simulink subsystem "ADC_Block"  (R2024b)
settings: Solver=VariableStepAuto  StartTime=0.0  StopTime=10.0  RelTol=1e-3
undefined symbols (not defined in the file or in its folder): circularBufferSize, samplingTime
settings Model: Creator=JesseJabezArendse  LastModifiedBy=JesseJabezArendse
settings RTWCC: GPUComputeCapability=3.5

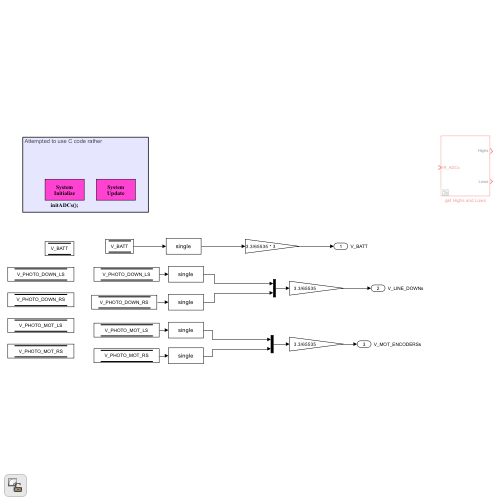
[thumbnail: Simulink's stored preview of the top-level diagram]
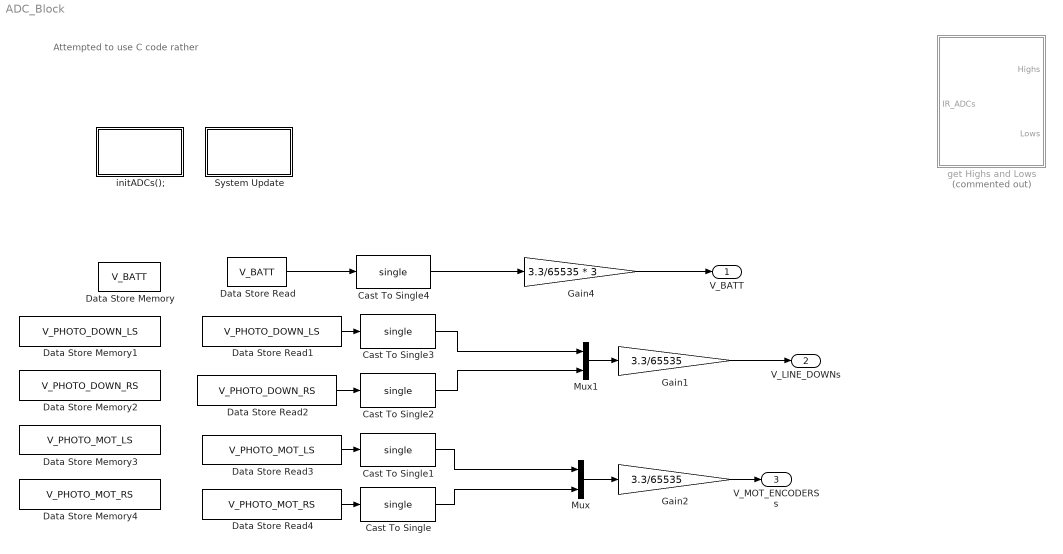
== system ADC_Block ==
  note: Attempted to use C code rather
  Cast To Single{,1..4} (5 alike) : DataTypeConversion  OutDataTypeStr=single  SaturateOnIntegerOverflow=off  RndMeth=Floor
  Data Store Memory : DataStoreMemory  DataStoreName=V_BATT  WriteAfterWriteMsg=warning  ShowAdditionalParam=off  OutDataTypeStr=uint16  Dimensions=1
  Data Store Memory1 : DataStoreMemory  DataStoreName=V_PHOTO_DOWN_LS  WriteAfterWriteMsg=warning  ShowAdditionalParam=off  OutDataTypeStr=uint16  Dimensions=1
  Data Store Memory2 : DataStoreMemory  DataStoreName=V_PHOTO_DOWN_RS  WriteAfterWriteMsg=warning  ShowAdditionalParam=off  OutDataTypeStr=uint16  Dimensions=1
  Data Store Memory3 : DataStoreMemory  DataStoreName=V_PHOTO_MOT_LS  WriteAfterWriteMsg=warning  ShowAdditionalParam=off  OutDataTypeStr=uint16  Dimensions=1
  Data Store Memory4 : DataStoreMemory  DataStoreName=V_PHOTO_MOT_RS  WriteAfterWriteMsg=warning  ShowAdditionalParam=off  OutDataTypeStr=uint16  Dimensions=1
  Data Store Read : DataStoreRead  DataStoreName=V_BATT  IndexOptions=Index vector (dialog)  Indices=1  OutputSizes=1
  Data Store Read1 : DataStoreRead  DataStoreName=V_PHOTO_DOWN_LS  IndexOptions=Index vector (dialog)  Indices=1  OutputSizes=1
  Data Store Read2 : DataStoreRead  DataStoreName=V_PHOTO_DOWN_RS  IndexOptions=Index vector (dialog)  Indices=1  OutputSizes=1
  Data Store Read3 : DataStoreRead  DataStoreName=V_PHOTO_MOT_LS  IndexOptions=Index vector (dialog)  Indices=1  OutputSizes=1
  Data Store Read4 : DataStoreRead  DataStoreName=V_PHOTO_MOT_RS  IndexOptions=Index vector (dialog)  Indices=1  OutputSizes=1
  Gain1 : Gain  Gain=3.3/65535
  Gain2 : Gain  Gain=3.3/65535
  Gain4 : Gain  Gain=3.3/65535 * 3
  Mux : Mux  Inputs=2
  Mux1 : Mux  Inputs=2
  System Update : Subsystem  mask(System Update){ShowInLibBrowser=0}
      mask prompts: ShowInLibBrowser "Simulink:masks:CustCodeMaskParam1_MP"
      settings: CopyFcn=cccopyfcn(gcb)  OpenFcn=ccopenfcn('System Update Function')
      mask Help: eval('feval(''rtwprivate'',''rtwhelpview'',''rtw_sys_update_block'')');
      mask Display: disp('System\nUpdate');
  get Highs and Lows : Subsystem  Commented=on
  initADCs(); : Subsystem  mask(System Initialize){ShowInLibBrowser=0}
      mask prompts: ShowInLibBrowser "Simulink:masks:CustCodeMaskParam1_MP"
      settings: CopyFcn=cccopyfcn(gcb)  OpenFcn=ccopenfcn('System Initialize Function')
      mask Help: eval('feval(''rtwprivate'',''rtwhelpview'',''rtw_sys_initialize_block'')');
      mask Display: disp('System\nInitialize');
  V_BATT : Outport
  V_LINE_DOWNs : Outport  Port=2
  V_MOT_ENCODERSs : Outport  Port=3
  wires:
  Mux1/1 -> Gain1/1
  Gain4/1 -> V_BATT/1
  Mux/1 -> Gain2/1
  Data Store Read/1 -> Cast To Single4/1
  Data Store Read3/1 -> Cast To Single1/1
  Data Store Read4/1 -> Cast To Single/1
  Data Store Read1/1 -> Cast To Single3/1
  Data Store Read2/1 -> Cast To Single2/1
  Gain1/1 -> V_LINE_DOWNs/1
  Gain2/1 -> V_MOT_ENCODERSs/1
  Cast To Single/1 -> Mux/2
  Cast To Single1/1 -> Mux/1
  Cast To Single2/1 -> Mux1/2
  Cast To Single3/1 -> Mux1/1
  Cast To Single4/1 -> Gain4/1

== system ADC_Block/System Update ==

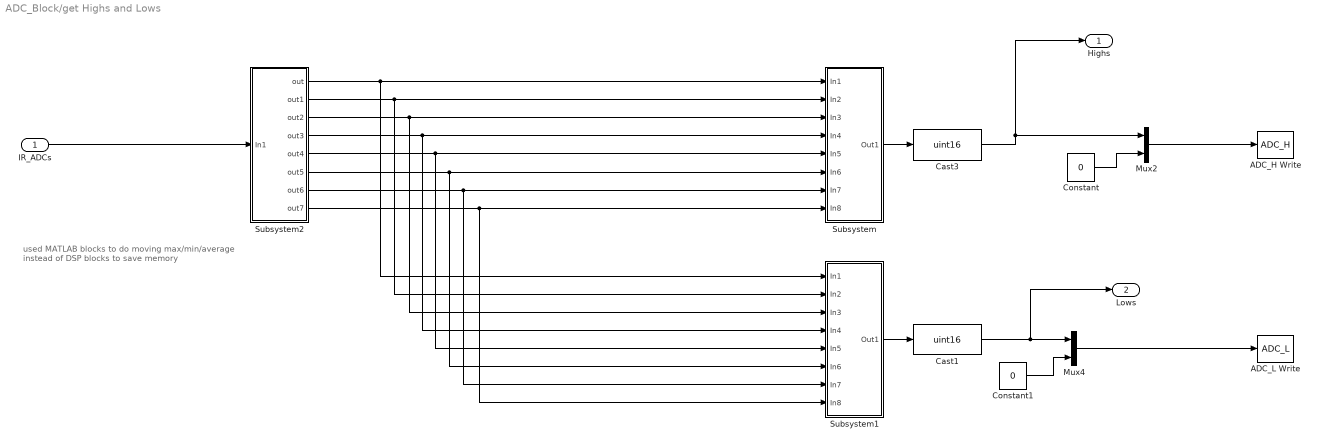
== system ADC_Block/get Highs and Lows ==
  note: used MATLAB blocks to do moving max/min/average
      | instead of DSP blocks to save memory
  IR_ADCs : Inport  PortDimensions=8  SampleTime=samplingTime
  ADC_H Write : DataStoreWrite  DataStoreName=ADC_H  SampleTime=samplingTime  IndexOptions=Index vector (dialog)  Indices=1  OutputSizes=1
  ADC_L Write : DataStoreWrite  DataStoreName=ADC_L  SampleTime=samplingTime  IndexOptions=Index vector (dialog)  Indices=1  OutputSizes=1
  Cast1 : DataTypeConversion  OutDataTypeStr=uint16  SaturateOnIntegerOverflow=off  RndMeth=Floor
  Cast3 : DataTypeConversion  OutDataTypeStr=uint16  SaturateOnIntegerOverflow=off  RndMeth=Floor
  Constant : Constant  Value=0  OutDataTypeStr=uint16  SampleTime=samplingTime
  Constant1 : Constant  Value=0  OutDataTypeStr=uint16  SampleTime=samplingTime
  Mux2 : Mux  Inputs=2
  Mux4 : Mux  Inputs=2
  Subsystem : Subsystem
  Subsystem1 : Subsystem
  Subsystem2 : Subsystem
  Highs : Outport
  Lows : Outport  Port=2
  wires:
  Cast3/1 -> Highs/1, Mux2/1
  Cast1/1 -> Mux4/1, Lows/1
  IR_ADCs/1 -> Subsystem2/1(In1)
  Subsystem2/3(out2) -> Subsystem1/3(In3), Subsystem/3(In3)
  Subsystem2/1(out) -> Subsystem/1(In1), Subsystem1/1(In1)
  Subsystem2/2(out1) -> Subsystem1/2(In2), Subsystem/2(In2)
  Subsystem2/4(out3) -> Subsystem1/4(In4), Subsystem/4(In4)
  Subsystem2/6(out5) -> Subsystem1/6(In6), Subsystem/6(In6)
  Subsystem2/7(out6) -> Subsystem1/7(In7), Subsystem/7(In7)
  Subsystem2/5(out4) -> Subsystem1/5(In5), Subsystem/5(In5)
  Subsystem2/8(out7) -> Subsystem1/8(In8), Subsystem/8(In8)
  Subsystem1/1(Out1) -> Cast1/1
  Subsystem/1(Out1) -> Cast3/1
  Mux4/1 -> ADC_L Write/1
  Mux2/1 -> ADC_H Write/1
  Constant1/1 -> Mux4/2
  Constant/1 -> Mux2/2

== system ADC_Block/initADCs(); ==

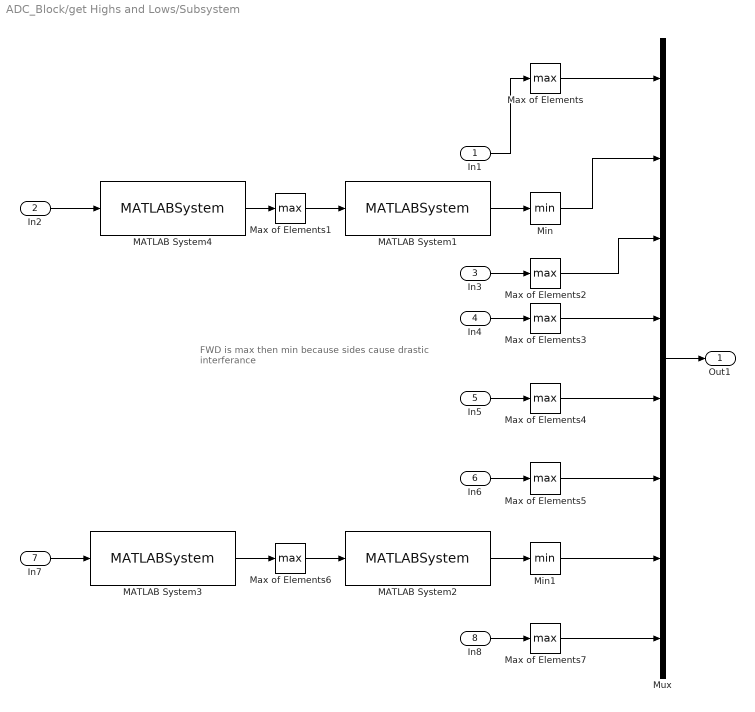
== system ADC_Block/get Highs and Lows/Subsystem ==
  note: FWD is max then min because sides cause drastic interferance
  In1 : Inport
  In2 : Inport  Port=2
  In3 : Inport  Port=3
  In4 : Inport  Port=4
  In5 : Inport  Port=5
  In6 : Inport  Port=6
  In7 : Inport  Port=7
  In8 : Inport  Port=8
  MATLAB System1 : MATLABSystem  System=CircularBuffer  BufferLength=circularBufferSize  InitialCondition=0  SimulateUsing=Code generation
      mask Type: CircularBuffer
      mask Display:
      | disp('CircularBuffer');
      | port_label('input',1,'signal');
      | port_label('output',1,'out');
  MATLAB System2 : MATLABSystem  System=CircularBuffer  BufferLength=circularBufferSize  InitialCondition=0  SimulateUsing=Code generation
      mask Type: CircularBuffer
      mask Display:
      | disp('CircularBuffer');
      | port_label('input',1,'signal');
      | port_label('output',1,'out');
  MATLAB System3 : MATLABSystem  System=CircularBuffer  BufferLength=circularBufferSize-15  InitialCondition=0  SimulateUsing=Code generation
      mask Type: CircularBuffer
      mask Display:
      | disp('CircularBuffer');
      | port_label('input',1,'signal');
      | port_label('output',1,'out');
  MATLAB System4 : MATLABSystem  System=CircularBuffer  BufferLength=circularBufferSize-15  InitialCondition=0  SimulateUsing=Code generation
      mask Type: CircularBuffer
      mask Display:
      | disp('CircularBuffer');
      | port_label('input',1,'signal');
      | port_label('output',1,'out');
  Max of Elements{,2..5,7} (6 alike) : MinMax  Function=max  OutDataTypeStr=uint16
  Max of Elements1 : MinMax  Function=max
  Max of Elements6 : MinMax  Function=max
  Min : MinMax  OutDataTypeStr=uint16
  Min1 : MinMax  OutDataTypeStr=uint16
  Mux : Mux  Inputs=8
  Out1 : Outport
  wires:
  Mux/1 -> Out1/1
  Max of Elements7/1 -> Mux/8
  Max of Elements5/1 -> Mux/6
  Max of Elements4/1 -> Mux/5
  Max of Elements3/1 -> Mux/4
  Max of Elements2/1 -> Mux/3
  Min/1 -> Mux/2
  Max of Elements/1 -> Mux/1
  In8/1 -> Max of Elements7/1
  MATLAB System2/1 -> Min1/1
  In6/1 -> Max of Elements5/1
  In4/1 -> Max of Elements3/1
  In3/1 -> Max of Elements2/1
  MATLAB System1/1 -> Min/1
  Max of Elements1/1 -> MATLAB System1/1
  Max of Elements6/1 -> MATLAB System2/1
  MATLAB System4/1 -> Max of Elements1/1
  Min1/1 -> Mux/7
  MATLAB System3/1 -> Max of Elements6/1
  In7/1 -> MATLAB System3/1
  In2/1 -> MATLAB System4/1
  In1/1 -> Max of Elements/1
  In5/1 -> Max of Elements4/1

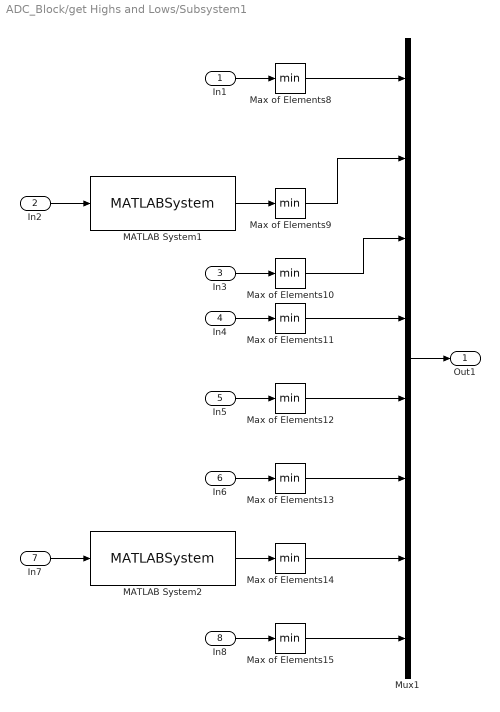
== system ADC_Block/get Highs and Lows/Subsystem1 ==
  In1 : Inport
  In2 : Inport  Port=2
  In3 : Inport  Port=3
  In4 : Inport  Port=4
  In5 : Inport  Port=5
  In6 : Inport  Port=6
  In7 : Inport  Port=7
  In8 : Inport  Port=8
  MATLAB System1 : MATLABSystem  System=CircularBuffer  BufferLength=circularBufferSize  InitialCondition=0  SimulateUsing=Code generation
      mask Type: CircularBuffer
      mask Display:
      | disp('CircularBuffer');
      | port_label('input',1,'signal');
      | port_label('output',1,'out');
  MATLAB System2 : MATLABSystem  System=CircularBuffer  BufferLength=circularBufferSize  InitialCondition=0  SimulateUsing=Code generation
      mask Type: CircularBuffer
      mask Display:
      | disp('CircularBuffer');
      | port_label('input',1,'signal');
      | port_label('output',1,'out');
  Max of Elements{8..15} (8 alike) : MinMax  OutDataTypeStr=uint16
  Mux1 : Mux  Inputs=8
  Out1 : Outport
  wires:
  Mux1/1 -> Out1/1
  Max of Elements13/1 -> Mux1/6
  Max of Elements11/1 -> Mux1/4
  Max of Elements10/1 -> Mux1/3
  Max of Elements9/1 -> Mux1/2
  Max of Elements8/1 -> Mux1/1
  In8/1 -> Max of Elements15/1
  MATLAB System2/1 -> Max of Elements14/1
  In3/1 -> Max of Elements10/1
  In7/1 -> MATLAB System2/1
  In4/1 -> Max of Elements11/1
  Max of Elements15/1 -> Mux1/8
  In5/1 -> Max of Elements12/1
  MATLAB System1/1 -> Max of Elements9/1
  In6/1 -> Max of Elements13/1
  In2/1 -> MATLAB System1/1
  Max of Elements14/1 -> Mux1/7
  In1/1 -> Max of Elements8/1
  Max of Elements12/1 -> Mux1/5

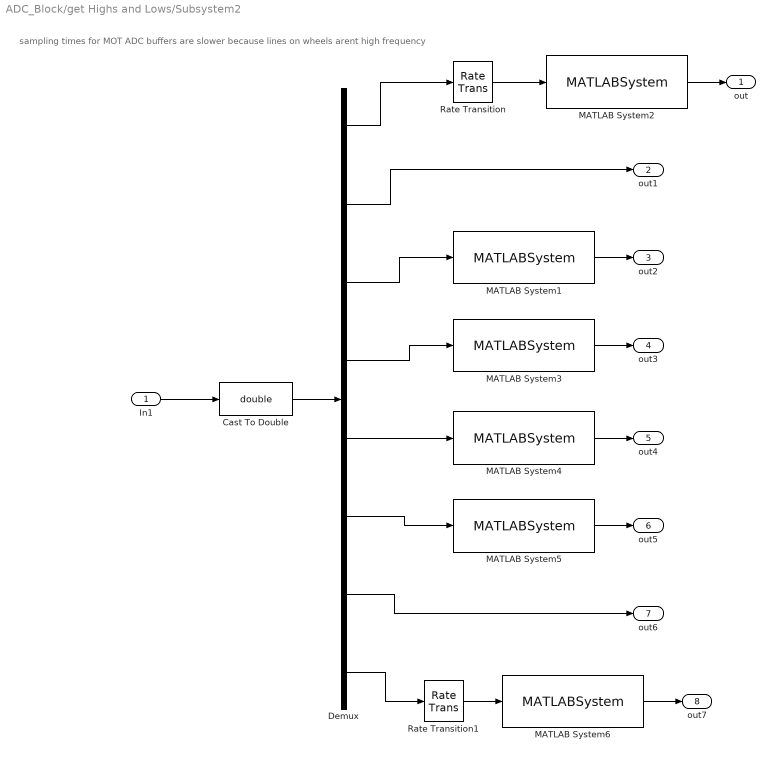
== system ADC_Block/get Highs and Lows/Subsystem2 ==
  note: sampling times for MOT ADC buffers are slower because lines on wheels arent high frequency
  In1 : Inport
  Cast To Double : DataTypeConversion  OutDataTypeStr=double  SaturateOnIntegerOverflow=off  RndMeth=Floor
  Demux : Demux  Outputs=8
  MATLAB System{1..6} (6 alike) : MATLABSystem  System=CircularBuffer  BufferLength=circularBufferSize  InitialCondition=0  SimulateUsing=Code generation
      mask Type: CircularBuffer
      mask Display:
      | disp('CircularBuffer');
      | port_label('input',1,'signal');
      | port_label('output',1,'out');
  Rate Transition : RateTransition  OutPortSampleTime=0.1
  Rate Transition1 : RateTransition  OutPortSampleTime=0.1
  out : Outport
  out1 : Outport  Port=2
  out2 : Outport  Port=3
  out3 : Outport  Port=4
  out4 : Outport  Port=5
  out5 : Outport  Port=6
  out6 : Outport  Port=7
  out7 : Outport  Port=8
  wires:
  Rate Transition1/1 -> MATLAB System6/1
  Rate Transition/1 -> MATLAB System2/1
  Demux/1 -> Rate Transition/1
  Cast To Double/1 -> Demux/1
  Demux/7 -> out6/1
  MATLAB System5/1 -> out5/1
  MATLAB System4/1 -> out4/1
  MATLAB System3/1 -> out3/1
  MATLAB System1/1 -> out2/1
  MATLAB System2/1 -> out/1
  Demux/8 -> Rate Transition1/1
  MATLAB System6/1 -> out7/1
  Demux/4 -> MATLAB System3/1
  Demux/2 -> out1/1
  Demux/3 -> MATLAB System1/1
  Demux/6 -> MATLAB System5/1
  Demux/5 -> MATLAB System4/1
  In1/1 -> Cast To Double/1
